simulink model "UART_communication"  (Simulink 7.8)
settings: Solver=FixedStepDiscrete  SolverMode=SingleTasking  StartTime=0.0  StopTime=inf  FixedStep=0.02  RelTol=1e-3
PreLoadFcn:
  | addpath([cd filesep 'QuadCom']);
InitFcn:
  | %cd('..\Uart_Com');
libraries: LIB_Quad_Com x2
settings Model: Creator=Michael  LastModifiedBy=erk
settings DebuggingCC: FcnCallInpInsideContextMsg=Use local settings  StrictBusMsg=Warning
settings HardwareCC: ProdLargestAtomicInteger=Long  ProdLargestAtomicFloat=Float  ProdHWDeviceType=ARM Compatible->ARM 7
settings SFSimCC: SimParseCustomCode=off

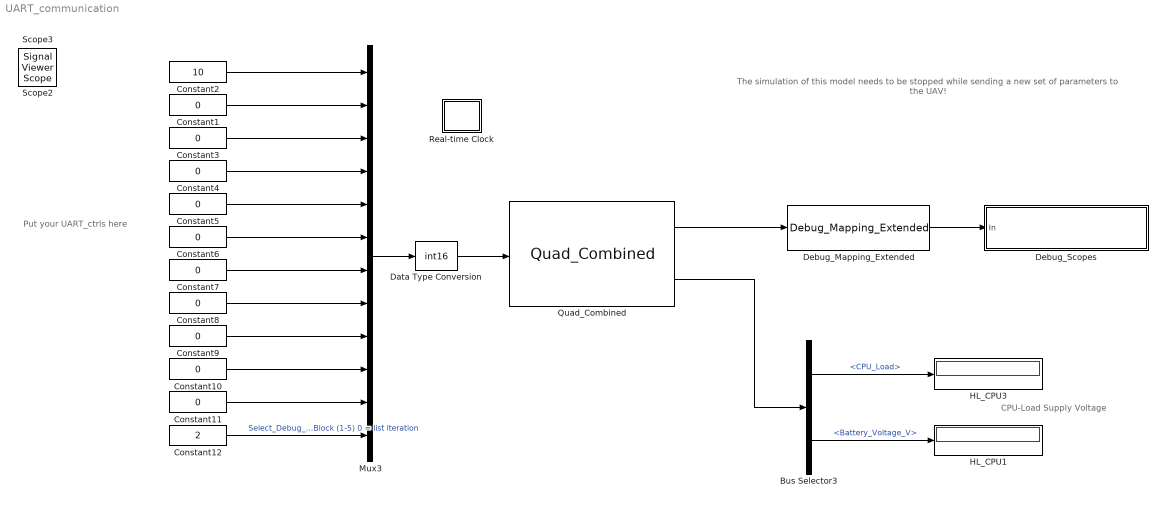
== system UART_communication ==
  note: CPU-Load
      |
      |
      |
      |
      | Supply Voltage
  note: The simulation of this model needs to be stopped while
      |  sending a new set of parameters to the UAV!
  note: Put your UART_ctrls here
  Bus Selector3 : BusSelector  OutputSignals=CPU_Load,Battery_Voltage_V
  Constant{1,3..11} (10 alike) : Constant  Value=0  VectorParams1D=off  OutDataTypeStr=fixdt(1,16,10)  SampleTime=0.02
  Constant12 : Constant  Value=2  VectorParams1D=off  OutDataTypeStr=fixdt(1,16,10)  SampleTime=0.02
  Constant2 : Constant  Value=10  VectorParams1D=off  OutDataTypeStr=fixdt(1,16,10)  SampleTime=0.02
  Data Type Conversion : DataTypeConversion  OutDataTypeStr=int16  ConvertRealWorld=Stored Integer (SI)
  Debug_Mapping_Extended : LIB_Quad_Com/Debug_Mapping_Extended
  Debug_Scopes : Subsystem
  HL_CPU1 : Display
  HL_CPU3 : Display
  Mux3 : Mux  Inputs=12
  Quad_Combined : LIB_Quad_Com/Quad_Combined  baudrate=57600
  Real-time Clock : Subsystem  mask(Real-time Clock){sample_time=0.02, tolerance=1}
      mask prompts: sample_time "Synchronize with real-time every n seconds:"; tolerance "Real-time warning tolerance (seconds):"
      mask help: Real-time Synchronization Block
      mask Help: This block synchronizes simulation time with the PC real-time clock or UNIX system clock. The first dialog entry is the period at which the clock is checked to insure real-time synchronization. The second dialog entry is the number of seconds that the simulation time must be within real-time before a warning is printed.
      mask Display: plot(0,0,100,100,[40,60,60,54,54,64,69,76,82,77,81,83,83,81,78,74,70,64,57,49,41,35,32,30,30,31,34,40,47,47,40,40],[90,90,85,85,80,79,76,87,80,70,64,57,49,41,33,28,24,22,21,23,25,31,37,46,56,65,73,78,80,85,85,90],[69,53,53],[64,50,73])
  Scope2 : SignalViewerScope  IOType=viewer  RefreshTime=0.035000
      settings: YMin=-0.09  YMax=0.07  SaveName=ScopeData2
  Scope3 : SignalViewerScope  IOType=viewer  RefreshTime=0.035000
      settings: YMin=-1.25  YMax=2.75  SaveName=ScopeData3
  wires:
  Quad_Combined/2 -> Bus Selector3/1
  Quad_Combined/1 -> Debug_Mapping_Extended/1
  Data Type Conversion/1 -> Quad_Combined/1
  Mux3/1 -> Data Type Conversion/1
  Constant2/1 -> Mux3/1
  Constant1/1 -> Mux3/2
  Constant3/1 -> Mux3/3
  Constant4/1 -> Mux3/4
  Constant5/1 -> Mux3/5
  Constant6/1 -> Mux3/6
  Constant7/1 -> Mux3/7
  Constant8/1 -> Mux3/8
  Constant9/1 -> Mux3/9
  Constant10/1 -> Mux3/10
  Constant11/1 -> Mux3/11
  Constant12/1 -> Mux3/12  "Select_Debug_Block (1-5) 0 = list iteration"
  Bus Selector3/1 -> HL_CPU3/1  "<CPU_Load>"
  Bus Selector3/2 -> HL_CPU1/1  "<Battery_Voltage_V>"
  Debug_Mapping_Extended/1 -> Debug_Scopes/1(In)

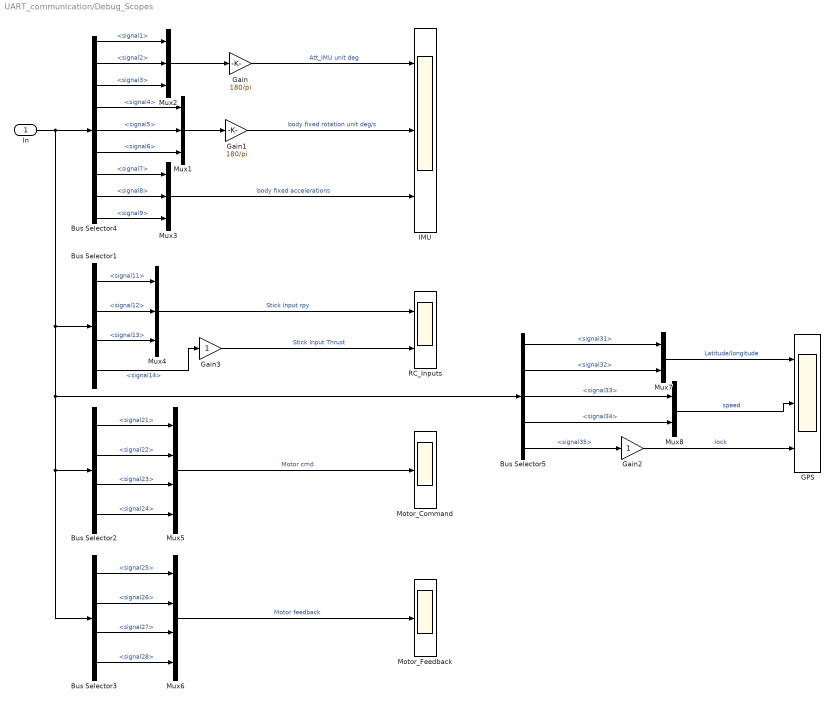
== system UART_communication/Debug_Scopes ==
  In : Inport
  Bus Selector1 : BusSelector  OutputSignals=signal11,signal12,signal13,signal14
  Bus Selector2 : BusSelector  OutputSignals=signal21,signal22,signal23,signal24
  Bus Selector3 : BusSelector  OutputSignals=signal25,signal26,signal27,signal28
  Bus Selector4 : BusSelector  OutputSignals=signal1,signal2,signal3,signal4,signal5,signal6,signal7,signal8,signal9
  Bus Selector5 : BusSelector  OutputSignals=signal31,signal32,signal33,signal34,signal35
  GPS : Scope  NumInputPorts=3
      settings: TimeRange=10  YMin=10~-1.2~-1  YMax=50~0.5~1
  Gain : Gain  Gain=180/pi
  Gain1 : Gain  Gain=180/pi
  Gain2 : Gain
  Gain3 : Gain
  IMU : Scope  NumInputPorts=3
      settings: TimeRange=3  YMin=-2.5~-1.25~-10  YMax=20~1.5~1  SaveName=ScopeData2
  Motor_Command : Scope
      settings: TimeRange=30  YMin=0  YMax=1  SaveName=ScopeData4
  Motor_Feedback : Scope
      settings: TimeRange=30  YMin=0  YMax=0.3
  Mux{1..4} (4 alike) : Mux  Inputs=3
  Mux5 : Mux
  Mux6 : Mux
  Mux7 : Mux  Inputs=2
  Mux8 : Mux  Inputs=2
  RC_Inputs : Scope  NumInputPorts=2
      settings: TimeRange=30  YMin=-1~-1  YMax=1~1  SaveName=ScopeData3
  wires:
  In/1 -> Bus Selector4/1, Bus Selector1/1, Bus Selector2/1, Bus Selector3/1, Bus Selector5/1
  Bus Selector4/1 -> Mux2/1  "<signal1>"
  Bus Selector4/2 -> Mux2/2  "<signal2>"
  Bus Selector4/3 -> Mux2/3  "<signal3>"
  Bus Selector4/4 -> Mux1/1  "<signal4>"
  Bus Selector4/5 -> Mux1/2  "<signal5>"
  Bus Selector4/6 -> Mux1/3  "<signal6>"
  Bus Selector4/7 -> Mux3/1  "<signal7>"
  Bus Selector4/8 -> Mux3/2  "<signal8>"
  Bus Selector4/9 -> Mux3/3  "<signal9>"
  Mux2/1 -> Gain/1
  Mux1/1 -> Gain1/1
  Mux3/1 -> IMU/3  "body fixed accelerations"
  Gain/1 -> IMU/1  "Att_IMU unit deg"
  Gain1/1 -> IMU/2  "body fixed rotation unit deg/s"
  Bus Selector1/1 -> Mux4/1  "<signal11>"
  Bus Selector1/2 -> Mux4/2  "<signal12>"
  Bus Selector1/3 -> Mux4/3  "<signal13>"
  Mux4/1 -> RC_Inputs/1  "Stick Input rpy"
  Bus Selector1/4 -> Gain3/1  "<signal14>"
  Gain3/1 -> RC_Inputs/2  "Stick Input Thrust"
  Bus Selector2/1 -> Mux5/1  "<signal21>"
  Bus Selector2/2 -> Mux5/2  "<signal22>"
  Bus Selector2/3 -> Mux5/3  "<signal23>"
  Bus Selector2/4 -> Mux5/4  "<signal24>"
  Mux5/1 -> Motor_Command/1  "Motor cmd"
  Bus Selector3/1 -> Mux6/1  "<signal25>"
  Bus Selector3/2 -> Mux6/2  "<signal26>"
  Bus Selector3/3 -> Mux6/3  "<signal27>"
  Bus Selector3/4 -> Mux6/4  "<signal28>"
  Mux6/1 -> Motor_Feedback/1  "Motor feedback"
  Mux7/1 -> GPS/1  "Latitude/longitude"
  Bus Selector5/1 -> Mux7/1  "<signal31>"
  Bus Selector5/2 -> Mux7/2  "<signal32>"
  Bus Selector5/3 -> Mux8/1  "<signal33>"
  Bus Selector5/4 -> Mux8/2  "<signal34>"
  Mux8/1 -> GPS/2  "speed"
  Bus Selector5/5 -> Gain2/1  "<signal35>"
  Gain2/1 -> GPS/3  "lock"

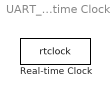
== system UART_communication/Real-time Clock ==
  Real-time Clock : S-Function  FunctionName=rtclock  Parameters=sample_time, tolerance  EnableBusSupport=off
